simulink model "lab2_2"  (R2014b)
settings: Solver=ode45  StartTime=0.0  StopTime=20  RelTol=1e-6
libraries: simulink x3
settings Model: Creator=StudentPA  LastModifiedBy=StudentPA

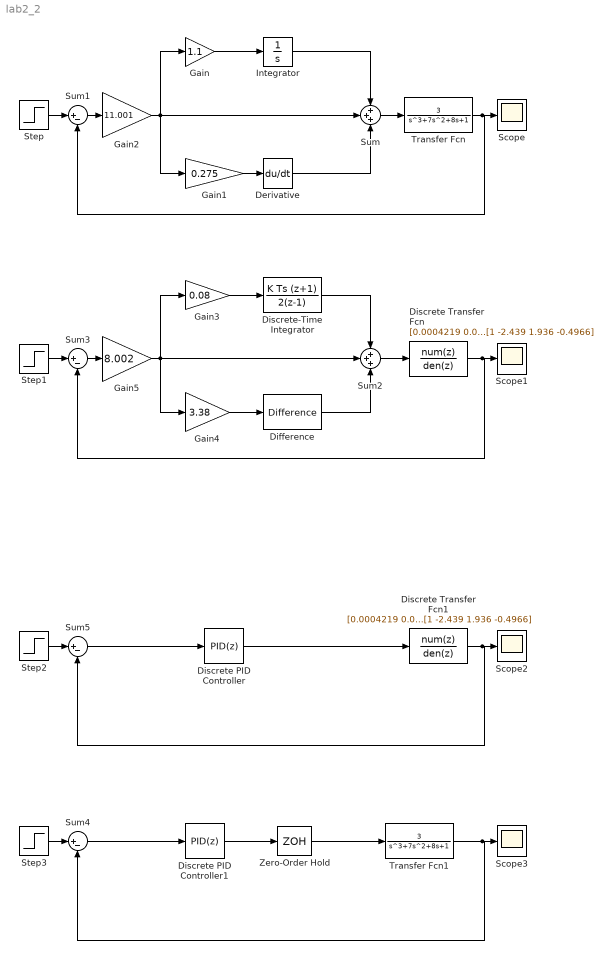
== system lab2_2 ==
  Derivative : Derivative
  Difference : simulink/Discrete/Difference  ICPrevInput=0.0  InputProcessing=Inherited  OutMin=[]  OutMax=[]  OutDataType=fixdt(1, 16)  OutScaling=2^-10  DoSatur=off
  Discrete Transfer Fcn : DiscreteTransferFcn  Numerator=[0.0004219 0.001424 0.0002974]  Denominator=[1 -2.439 1.936 -0.4966]  SampleTime=1
  Discrete Transfer Fcn1 : DiscreteTransferFcn  Numerator=[0.0004219 0.001424 0.0002974]  Denominator=[1 -2.439 1.936 -0.4966]  SampleTime=1
  Discrete PID Controller : simulink/Continuous/PID Controller  Controller=PID  TimeDomain=Discrete-time  SampleTime=1  IntegratorMethod=Trapezoidal  FilterMethod=Trapezoidal  Form=Ideal  P=2.36166332284011  I=0.0082012902823336  D=5.40743903182152  N=0.283992931240168  InitialConditionSource=internal  InitialConditionForIntegrator=0  InitialConditionForFilter=0  ExternalReset=none  LimitOutput=off  UpperSaturationLimit=inf  LowerSaturationLimit=-inf  LinearizeAsGain=off  AntiWindupMode=none  Kb=1  TrackingMode=off  Kt=1  PParamMin=[]  PParamMax=[]  IParamMin=[]  IParamMax=[]  DParamMin=[]  DParamMax=[]  NParamMin=[]  NParamMax=[]  KbParamMin=[]  KbParamMax=[]  KtParamMin=[]  KtParamMax=[]  POutMin=[]  POutMax=[]  IOutMin=[]  IOutMax=[]  DOutMin=[]  DOutMax=[]  NOutMin=[]  NOutMax=[]  KbOutMin=[]  KbOutMax=[]  KtOutMin=[]  KtOutMax=[]  IntegratorOutMin=[]  IntegratorOutMax=[]  FilterOutMin=[]  FilterOutMax=[]  SumOutMin=[]  SumOutMax=[]  SumI1OutMin=[]  SumI1OutMax=[]  SumI2OutMin=[]  SumI2OutMax=[]  SumI3OutMin=[]  SumI3OutMax=[]  SumDOutMin=[]  SumDOutMax=[]  SaturationOutMin=[]  SaturationOutMax=[]  IntegratorContinuousStateAttributes=''  IntegratorStateMustResolveToSignalObject=off  IntegratorRTWStateStorageClass=Auto  FilterContinuousStateAttributes=''  FilterStateMustResolveToSignalObject=off  FilterRTWStateStorageClass=Auto  DifferentiatorICPrevScaledInput=0  DifferentiatorOutMin=[]  DifferentiatorOutMax=[]  UseFilter=on
  Discrete PID Controller1 : simulink/Continuous/PID Controller  Controller=PID  TimeDomain=Discrete-time  SampleTime=1  IntegratorMethod=Trapezoidal  FilterMethod=Trapezoidal  Form=Ideal  P=2.36166332284011  I=0.0082012902823336  D=5.40743903182152  N=0.283992931240168  InitialConditionSource=internal  InitialConditionForIntegrator=0  InitialConditionForFilter=0  ExternalReset=none  LimitOutput=off  UpperSaturationLimit=inf  LowerSaturationLimit=-inf  LinearizeAsGain=off  AntiWindupMode=none  Kb=1  TrackingMode=off  Kt=1  PParamMin=[]  PParamMax=[]  IParamMin=[]  IParamMax=[]  DParamMin=[]  DParamMax=[]  NParamMin=[]  NParamMax=[]  KbParamMin=[]  KbParamMax=[]  KtParamMin=[]  KtParamMax=[]  POutMin=[]  POutMax=[]  IOutMin=[]  IOutMax=[]  DOutMin=[]  DOutMax=[]  NOutMin=[]  NOutMax=[]  KbOutMin=[]  KbOutMax=[]  KtOutMin=[]  KtOutMax=[]  IntegratorOutMin=[]  IntegratorOutMax=[]  FilterOutMin=[]  FilterOutMax=[]  SumOutMin=[]  SumOutMax=[]  SumI1OutMin=[]  SumI1OutMax=[]  SumI2OutMin=[]  SumI2OutMax=[]  SumI3OutMin=[]  SumI3OutMax=[]  SumDOutMin=[]  SumDOutMax=[]  SaturationOutMin=[]  SaturationOutMax=[]  IntegratorContinuousStateAttributes=''  IntegratorStateMustResolveToSignalObject=off  IntegratorRTWStateStorageClass=Auto  FilterContinuousStateAttributes=''  FilterStateMustResolveToSignalObject=off  FilterRTWStateStorageClass=Auto  DifferentiatorICPrevScaledInput=0  DifferentiatorOutMin=[]  DifferentiatorOutMax=[]  UseFilter=on
  Discrete-Time Integrator : DiscreteIntegrator  IntegratorMethod=Integration: Trapezoidal  InitialConditionSetting=State (most efficient)
  Gain : Gain  Gain=1.1
  Gain1 : Gain  Gain=0.275
  Gain2 : Gain  Gain=11.001
  Gain3 : Gain  Gain=0.08
  Gain4 : Gain  Gain=3.38
  Gain5 : Gain  Gain=8.002  SampleTime=1
  Integrator : Integrator
  Scope{,1..3} (4 alike) : Scope
      Scope settings: YMin=0  YMax=2
      Scope1 settings: YMin=0  YMax=2
      Scope2 settings: YMin=0  YMax=2  SaveName=ScopeData2
      Scope3 settings: YMin=0  YMax=2  SaveName=ScopeData3
  Step{,1..3} (4 alike) : Step  Time=0  SampleTime=0
  Sum : Sum  Inputs=+++
  Sum{1,3..5} (4 alike) : Sum  Inputs=|+-
  Sum2 : Sum  Inputs=+++
  Transfer Fcn : TransferFcn  Numerator=[3]  Denominator=[1 7 8 1]
  Transfer Fcn1 : TransferFcn  Numerator=[3]  Denominator=[1 7 8 1]
  Zero-Order Hold : ZeroOrderHold
  wires:
  Sum/1 -> Transfer Fcn/1
  Step/1 -> Sum1/1
  Sum1/1 -> Gain2/1
  Gain2/1 -> Gain1/1, Sum/2, Gain/1
  Gain/1 -> Integrator/1
  Gain1/1 -> Derivative/1
  Integrator/1 -> Sum/1
  Derivative/1 -> Sum/3
  Transfer Fcn/1 -> Sum1/2, Scope/1
  Sum2/1 -> Discrete Transfer Fcn/1
  Step1/1 -> Sum3/1
  Sum3/1 -> Gain5/1
  Gain5/1 -> Gain4/1, Sum2/2, Gain3/1
  Gain3/1 -> Discrete-Time Integrator/1
  Gain4/1 -> Difference/1
  Discrete-Time Integrator/1 -> Sum2/1
  Difference/1 -> Sum2/3
  Discrete Transfer Fcn/1 -> Sum3/2, Scope1/1
  Step2/1 -> Sum5/1
  Sum5/1 -> Discrete PID Controller/1
  Discrete Transfer Fcn1/1 -> Sum5/2, Scope2/1
  Discrete PID Controller/1 -> Discrete Transfer Fcn1/1
  Step3/1 -> Sum4/1
  Transfer Fcn1/1 -> Sum4/2, Scope3/1
  Sum4/1 -> Discrete PID Controller1/1
  Discrete PID Controller1/1 -> Zero-Order Hold/1
  Zero-Order Hold/1 -> Transfer Fcn1/1
